simulink model "L0701"  (Simulink 9.1)
settings: Solver=FixedStepDiscrete  StartTime=0.0  StopTime=20  FixedStep=1  RelTol=1e-3
InitFcn:
  | inpdata
StopFcn:
  | result
settings Model: Creator=Asus  LastModifiedBy=Asus
settings DataIOCC: LimitDataPoints=on  MaxDataPoints=1  LoadExternalInput=on  SignalLogging=off  DSMLogging=off  SaveTime=off
settings OptimizationCC: LifeSpan=auto
settings DebuggingCC: UnderspecifiedInitializationDetection=Simplified  MergeDetectMultiDrivingBlocksExec=error  SFUnexpectedBacktrackingDiag=error  SFNoUnconditionalDefaultTransitionDiag=error  SFExecutionAtInitializationDiag=warning
settings HardwareCC: ProdBitPerPointer=64  ProdBitPerSizeT=64  ProdBitPerPtrDiffT=64  ProdLargestAtomicFloat=Float  ProdIntDivRoundTo=Zero  ProdEndianess=LittleEndian  ProdWordSize=64  ProdHWDeviceType=Intel->x86-64 (Windows64)
settings ModelReferenceCC: PropagateSignalLabelsOutOfModel=on
settings CodeAppCC: StateflowObjectComments=off
settings GRTTargetCC: TargetLangStandard=C99 (ISO)  CombineOutputUpdateFcns=on  GRTInterface=off
settings ConfigComp: CovMetricSettings=dwe  CovHtmlReporting=off  CovSaveCumulativeToWorkspaceVar=off  CovSaveSingleToWorkspaceVar=off  CovExternalEMLEnable=on

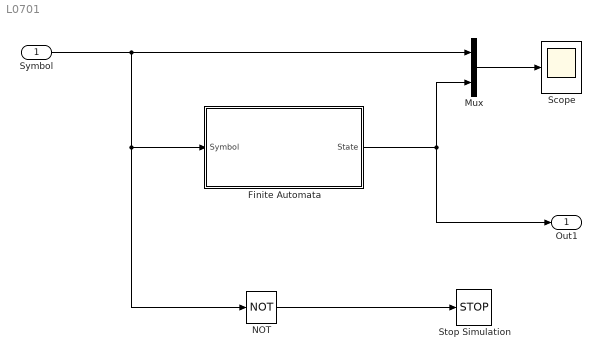
== system L0701 ==
  Symbol : Inport  OutDataTypeStr=double  SampleTime=1
  "Finite Automata " : Stateflow chart  TreatAsAtomicUnit=on
  Mux : Mux  Inputs=2
  NOT : Logic  Operator=NOT  AllPortsSameDT=off  OutDataTypeStr=boolean
  Scope : Scope
      settings: AttributesFormatString=[%<YMin>,%<YMax>]
  Stop Simulation : Stop
  Out1 : Outport  OutDataTypeStr=double
  wires:
  Symbol/1 -> NOT/1, "Finite Automata "/1(Symbol), Mux/1
  NOT/1 -> Stop Simulation/1
  Mux/1 -> Scope/1
  "Finite Automata "/1(State) -> Out1/1, Mux/2

== stateflow chart Finite Automata  ==
  state Zero
    entry:State=0;
  state First
    entry:State=-1;
  Zero -> First : [Symbol==1]
  (default) -> Zero
  First -> Zero [order 2] : [Symbol==1]
  First -> Zero [order 1] : [Symbol==2]
  data: State output double; Symbol input double
